simulink model "controller_sim"  (R2024a)
settings: Solver=FixedStepAuto  StartTime=0.0  StopTime=500  FixedStep=0.001  RelTol=1e-2
settings Model: Creator=filip  LastModifiedBy=raden
settings SolverCC: ZeroCrossAlgorithm=Adaptive
settings DebuggingCC: IgnoredZcDiagnostic=none

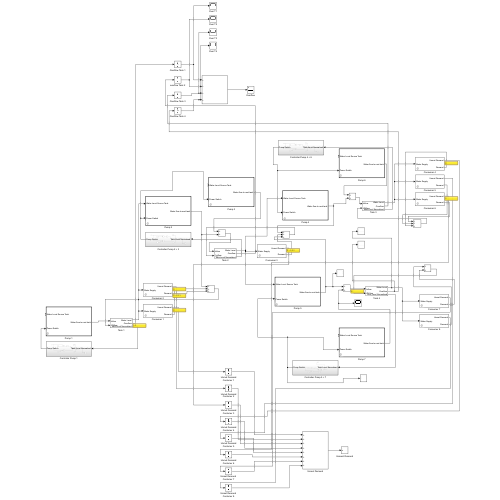
[thumbnail: Simulink's stored preview of the top-level diagram]
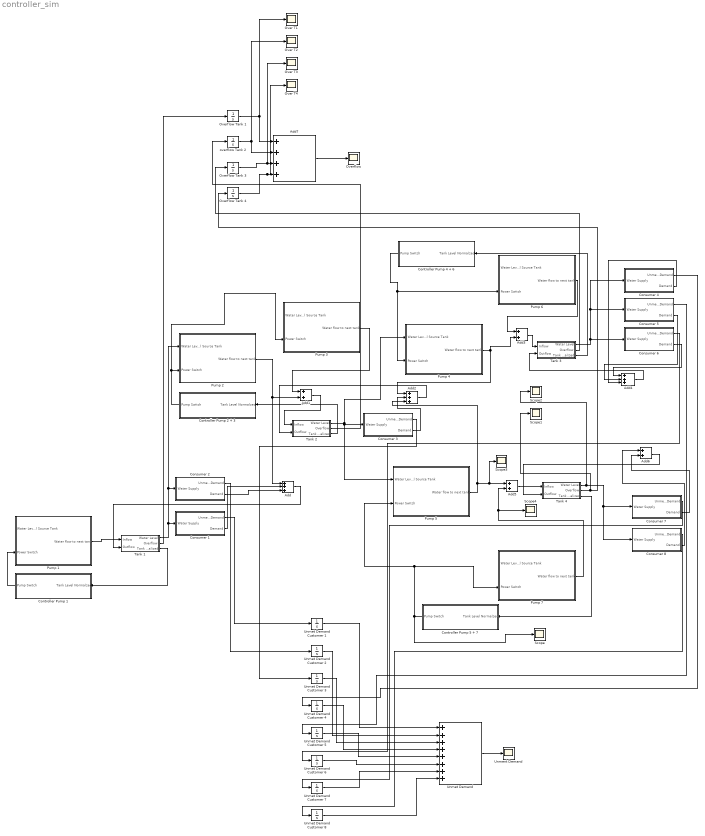
== system controller_sim ==
  Add : Sum  Inputs=+++
  Add{1,3,5..6} (4 alike) : Sum
  Add2 : Sum  Inputs=+++
  Add4 : Sum  Inputs=+++
  Add7 : Sum  Inputs=++++
  Consumer 1 : Subsystem  mask{a_i=3.0, f_i=0.4, d_i=2.0}
      mask prompts: f_i "frequenz"; d_i "delay"
  Consumer 2 : Subsystem  mask{a_i=8.0, f_i=0.6, d_i=0.5}
      mask prompts: f_i "frequenz"; d_i "delay"
  Consumer 3 : Subsystem  mask{a_i=5.0, f_i=0.2, d_i=4.0}
      mask prompts: f_i "frequenz"; d_i "delay"
  Consumer 4 : Subsystem  mask{a_i=5.0, f_i=1.0, d_i=3.0}
      mask prompts: f_i "frequenz"; d_i "delay"
  Consumer 5 : Subsystem  mask{a_i=2.0, f_i=0.4, d_i=4.0}
      mask prompts: f_i "frequenz"; d_i "delay"
  Consumer 6 : Subsystem  mask{a_i=7.0, f_i=0.1, d_i=5.0}
      mask prompts: f_i "frequenz"; d_i "delay"
  Consumer 7 : Subsystem  mask{a_i=2.0, f_i=0.9, d_i=7.0}
      mask prompts: f_i "frequenz"; d_i "delay"
  Consumer 8 : Subsystem  mask{a_i=5.0, f_i=0.6, d_i=4.0}
      mask prompts: f_i "frequenz"; d_i "delay"
  Controller Pump 1 : Subsystem
      settings: PortSchema="{\"entries\":[{\"content\":{\"sides\":[{\"content\":{\"connectorIds\":[\"Out1\"]},\"type\":\"ConnectorPlacement.EquallySpacedRectSide\",\"uuid\":\"c01aea8f-3a50-48ff-9d85-da287ef4ecfe\"},{\"content\":{\"connectorIds\":[\"In1\"],\"side\":\"RIGHT\"},\"type\":\"ConnectorPlacement.EquallySpacedRectSide\",\"uuid\":\"7272fdb4-8195-4269-b45d-955a00b5f153\"},{\"content\":{\"side\":\"TOP\"},\"type\":\"ConnectorPlacement.EquallySpacedRectSide\",\"uuid\":\"ead61a79-0064-4486-848a-5274f34ed301\"}]},\"type\":\"ConnectorPlacement.EquallySpacedConnector\",\"uuid\":\"31fbb0a2-b36d-48d4-9bb2-4bba902ab975\"}],\"packageUris\":[\"http://schema.mathworks.com/mf0/Connector/R2020b\"],\"version\":\"1.0\"}"
  Controller Pump 2 + 3 : Subsystem
      settings: PortSchema="{\"entries\":[{\"content\":{\"sides\":[{\"content\":{\"connectorIds\":[\"Out1\"]},\"type\":\"ConnectorPlacement.EquallySpacedRectSide\",\"uuid\":\"c01aea8f-3a50-48ff-9d85-da287ef4ecfe\"},{\"content\":{\"connectorIds\":[\"In1\"],\"side\":\"RIGHT\"},\"type\":\"ConnectorPlacement.EquallySpacedRectSide\",\"uuid\":\"7272fdb4-8195-4269-b45d-955a00b5f153\"},{\"content\":{\"side\":\"TOP\"},\"type\":\"ConnectorPlacement.EquallySpacedRectSide\",\"uuid\":\"ead61a79-0064-4486-848a-5274f34ed301\"}]},\"type\":\"ConnectorPlacement.EquallySpacedConnector\",\"uuid\":\"31fbb0a2-b36d-48d4-9bb2-4bba902ab975\"}],\"packageUris\":[\"http://schema.mathworks.com/mf0/Connector/R2020b\"],\"version\":\"1.0\"}"
  Controller Pump 4 + 6 : Subsystem
      settings: PortSchema="{\"entries\":[{\"content\":{\"sides\":[{\"content\":{\"connectorIds\":[\"Out1\"]},\"type\":\"ConnectorPlacement.EquallySpacedRectSide\",\"uuid\":\"c01aea8f-3a50-48ff-9d85-da287ef4ecfe\"},{\"content\":{\"connectorIds\":[\"In1\"],\"side\":\"RIGHT\"},\"type\":\"ConnectorPlacement.EquallySpacedRectSide\",\"uuid\":\"7272fdb4-8195-4269-b45d-955a00b5f153\"},{\"content\":{\"side\":\"TOP\"},\"type\":\"ConnectorPlacement.EquallySpacedRectSide\",\"uuid\":\"ead61a79-0064-4486-848a-5274f34ed301\"}]},\"type\":\"ConnectorPlacement.EquallySpacedConnector\",\"uuid\":\"31fbb0a2-b36d-48d4-9bb2-4bba902ab975\"}],\"packageUris\":[\"http://schema.mathworks.com/mf0/Connector/R2020b\"],\"version\":\"1.0\"}"
  Controller Pump 5 + 7 : Subsystem
      settings: PortSchema="{\"entries\":[{\"content\":{\"sides\":[{\"content\":{\"connectorIds\":[\"Out1\"]},\"type\":\"ConnectorPlacement.EquallySpacedRectSide\",\"uuid\":\"c01aea8f-3a50-48ff-9d85-da287ef4ecfe\"},{\"content\":{\"connectorIds\":[\"In1\"],\"side\":\"RIGHT\"},\"type\":\"ConnectorPlacement.EquallySpacedRectSide\",\"uuid\":\"7272fdb4-8195-4269-b45d-955a00b5f153\"},{\"content\":{\"side\":\"TOP\"},\"type\":\"ConnectorPlacement.EquallySpacedRectSide\",\"uuid\":\"ead61a79-0064-4486-848a-5274f34ed301\"}]},\"type\":\"ConnectorPlacement.EquallySpacedConnector\",\"uuid\":\"31fbb0a2-b36d-48d4-9bb2-4bba902ab975\"}],\"packageUris\":[\"http://schema.mathworks.com/mf0/Connector/R2020b\"],\"version\":\"1.0\"}"
  Over T{1..4} (4 alike) : Scope
  Overflow : Scope
  Overflow Tank 1 : Integrator
  Overflow Tank 3 : Integrator
  Overflow Tank 4 : Integrator
  Pump 1 : Subsystem  TreatAsAtomicUnit=on  mask{p_i=15}
      mask prompts: p_i "volume per Time (p_i)"
  Pump 2 : Subsystem  TreatAsAtomicUnit=on  mask{p_i=20}
      mask prompts: p_i "volume per Time (p_i)"
  Pump 3 : Subsystem  TreatAsAtomicUnit=on  mask{p_i=5}
      mask prompts: p_i "volume per Time (p_i)"
  Pump 4 : Subsystem  TreatAsAtomicUnit=on  mask{p_i=7}
      mask prompts: p_i "volume per Time (p_i)"
  Pump 5 : Subsystem  TreatAsAtomicUnit=on  mask{p_i=3}
      mask prompts: p_i "volume per Time (p_i)"
  Pump 6 : Subsystem  TreatAsAtomicUnit=on  mask{p_i=5}
      mask prompts: p_i "volume per Time (p_i)"
  Pump 7 : Subsystem  TreatAsAtomicUnit=on  mask{p_i=5}
      mask prompts: p_i "volume per Time (p_i)"
  Scope{,1..4} (5 alike) : Scope
  Tank 1 : Subsystem  mask{c_i=100, c_i_init=50}
      mask prompts: c_i "capacity (c_i)"; c_i_init "Init capacity (c_i_init)"
  Tank 2 : Subsystem  mask{c_i=100, c_i_init=50}
      mask prompts: c_i "capacity (c_i)"; c_i_init "Init capacity (c_i_init)"
  Tank 3 : Subsystem  mask{c_i=100, c_i_init=50}
      mask prompts: c_i "capacity (c_i)"; c_i_init "Init capacity (c_i_init)"
  Tank 4 : Subsystem  mask{c_i=100, c_i_init=0}
      mask prompts: c_i "capacity (c_i)"; c_i_init "Init capacity (c_i_init)"
  Unment Demand : Scope
  Unmet Demand : Sum  Inputs=++++++++
  Unmet Demand Customer {1..8} (8 alike) : Integrator
  overflow Tank 2 : Integrator
  wires:
  Pump 1/1(Water flow to next tank) -> Tank 1/1(Inflow)
  Add/1 -> Tank 1/2(Outflow)
  Tank 1/1(Water Level) -> Pump 2/1(Water Level Source Tank), Consumer 2/1(Water Supply), Consumer 1/1(Water Supply)
  Pump 2/1(Water flow to next tank) -> Add/1, Add1/2
  Pump 3/1(Water flow to next tank) -> Add1/1
  Add1/1 -> Tank 2/1(Inflow)
  Tank 2/1(Water Level) -> Consumer 3/1(Water Supply), Pump 5/1(Water Level Source Tank), Pump 4/1(Water Level Source Tank)
  Pump 4/1(Water flow to next tank) -> Add3/2, Add2/1
  Consumer 3/2(Demand) -> Add2/2
  Pump 5/1(Water flow to next tank) -> Add2/3, Scope3/1, Add5/1
  Add2/1 -> Tank 2/2(Outflow)
  Pump 6/1(Water flow to next tank) -> Add3/1
  Add3/1 -> Tank 3/1(Inflow)
  Tank 3/1(Water Level) -> Consumer 6/1(Water Supply), Consumer 5/1(Water Supply), Consumer 4/1(Water Supply)
  Consumer 6/2(Demand) -> Add4/1
  Consumer 5/2(Demand) -> Add4/2
  Consumer 4/2(Demand) -> Add4/3
  Add4/1 -> Tank 3/2(Outflow)
  Pump 7/1(Water flow to next tank) -> Add5/2, Scope4/1
  Add5/1 -> Tank 4/1(Inflow)
  Tank 4/1(Water Level) -> Scope2/1, Consumer 8/1(Water Supply), Consumer 7/1(Water Supply)
  Consumer 7/2(Demand) -> Add6/2
  Consumer 8/2(Demand) -> Add6/1
  Add6/1 -> Tank 4/2(Outflow)
  Consumer 2/1(Unmet Demand) -> Unmet Demand Customer 2/1
  Consumer 3/1(Unmet Demand) -> Unmet Demand Customer 3/1
  Consumer 4/1(Unmet Demand) -> Unmet Demand Customer 4/1
  Consumer 5/1(Unmet Demand) -> Unmet Demand Customer 5/1
  Consumer 6/1(Unmet Demand) -> Unmet Demand Customer 6/1
  Consumer 7/1(Unmet Demand) -> Unmet Demand Customer 7/1
  Consumer 8/1(Unmet Demand) -> Unmet Demand Customer 8/1
  Unmet Demand/1 -> Unment Demand/1
  Tank 1/2(Overflow) -> Overflow Tank 1/1
  Tank 2/2(Overflow) -> overflow Tank 2/1
  Tank 3/2(Overflow) -> Overflow Tank 3/1
  Tank 4/2(Overflow) -> Scope1/1, Overflow Tank 4/1
  Add7/1 -> Overflow/1
  Consumer 1/1(Unmet Demand) -> Unmet Demand Customer 1/1
  Consumer 1/2(Demand) -> Add/2
  Consumer 2/2(Demand) -> Add/3
  Overflow Tank 1/1 -> Over T1/1, Add7/1
  overflow Tank 2/1 -> Over T2/1, Add7/2
  Overflow Tank 3/1 -> Over T3/1, Add7/3
  Overflow Tank 4/1 -> Over T4/1, Add7/4
  Unmet Demand Customer 1/1 -> Unmet Demand/1
  Unmet Demand Customer 2/1 -> Unmet Demand/2
  Unmet Demand Customer 3/1 -> Unmet Demand/3
  Unmet Demand Customer 4/1 -> Unmet Demand/4
  Unmet Demand Customer 5/1 -> Unmet Demand/5
  Unmet Demand Customer 6/1 -> Unmet Demand/6
  Unmet Demand Customer 7/1 -> Unmet Demand/7
  Unmet Demand Customer 8/1 -> Unmet Demand/8
  Tank 1/3(Tank Level Normalized) -> Controller Pump 1/1(Tank Level Normalzed)
  Controller Pump 1/1(Pump Switch) -> Pump 1/2(Power Switch)
  Tank 2/3(Tank Level Normalized) -> Controller Pump 2 + 3/1(Tank Level Normalzed)
  Controller Pump 2 + 3/1(Pump Switch) -> Pump 2/2(Power Switch), Pump 3/2(Power Switch)
  Tank 3/3(Tank Level Normalized) -> Controller Pump 4 + 6/1(Tank Level Normalzed)
  Controller Pump 4 + 6/1(Pump Switch) -> Pump 4/2(Power Switch), Pump 6/2(Power Switch)
  Controller Pump 5 + 7/1(Pump Switch) -> Scope/1, Pump 7/2(Power Switch), Pump 5/2(Power Switch)
  Tank 4/3(Tank Level Normalized) -> Controller Pump 5 + 7/1(Tank Level Normalzed)

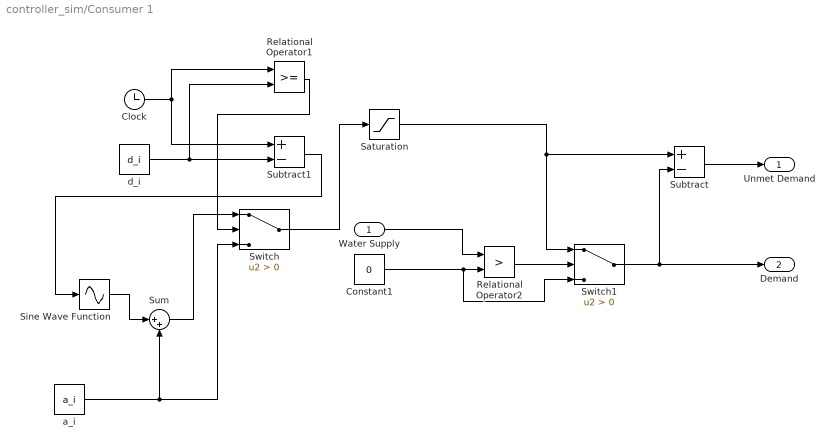
== system controller_sim/Consumer 1 ==
  Water Supply : Inport
  Clock : Clock
  Constant1 : Constant  Value=0
  Relational Operator1 : RelationalOperator  OutDataTypeStr=boolean  RndMeth=Simplest  InputSameDT=off
  Relational Operator2 : RelationalOperator  Operator=>  OutDataTypeStr=boolean  RndMeth=Simplest  InputSameDT=off
  Saturation : Saturate  UpperLimit=inf  LowerLimit=0
  Sine Wave Function : Sin  TimeSource=Use external signal  Amplitude=a_i  Frequency=f_i  SampleTime=0
  Subtract : Sum  Inputs=+-
  Subtract1 : Sum  Inputs=+-
  Sum : Sum  Inputs=|++
  Switch : Switch  Criteria=u2 > Threshold  SaturateOnIntegerOverflow=off  InputSameDT=off
  Switch1 : Switch  Criteria=u2 > Threshold  SaturateOnIntegerOverflow=off  InputSameDT=off
  a_i : Constant  Value=a_i
  d_i : Constant  Value=d_i
  Unmet Demand : Outport
  Demand : Outport  Port=2
  wires:
  a_i/1 -> Sum/2, Switch/3
  Switch/1 -> Saturation/1
  Saturation/1 -> Subtract/1, Switch1/1
  Clock/1 -> Relational Operator1/1, Subtract1/1
  d_i/1 -> Relational Operator1/2, Subtract1/2
  Subtract1/1 -> Sine Wave Function/1
  Relational Operator1/1 -> Switch/2
  Sum/1 -> Switch/1
  Sine Wave Function/1 -> Sum/1
  Water Supply/1 -> Relational Operator2/1
  Constant1/1 -> Relational Operator2/2, Switch1/3
  Relational Operator2/1 -> Switch1/2
  Switch1/1 -> Subtract/2, Demand/1
  Subtract/1 -> Unmet Demand/1

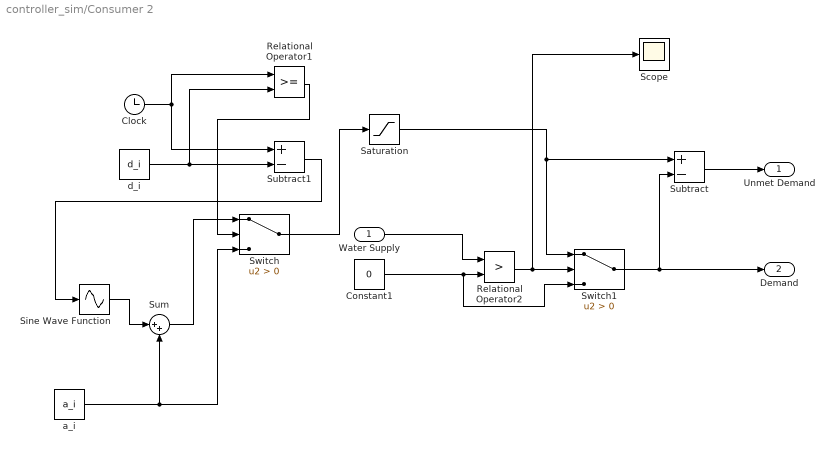
== system controller_sim/Consumer 2 ==
  Water Supply : Inport
  Clock : Clock
  Constant1 : Constant  Value=0
  Relational Operator1 : RelationalOperator  OutDataTypeStr=boolean  RndMeth=Simplest  InputSameDT=off
  Relational Operator2 : RelationalOperator  Operator=>  OutDataTypeStr=boolean  RndMeth=Simplest  InputSameDT=off
  Saturation : Saturate  UpperLimit=inf  LowerLimit=0
  Scope : Scope
  Sine Wave Function : Sin  TimeSource=Use external signal  Amplitude=a_i  Frequency=f_i  SampleTime=0
  Subtract : Sum  Inputs=+-
  Subtract1 : Sum  Inputs=+-
  Sum : Sum  Inputs=|++
  Switch : Switch  Criteria=u2 > Threshold  SaturateOnIntegerOverflow=off  InputSameDT=off
  Switch1 : Switch  Criteria=u2 > Threshold  SaturateOnIntegerOverflow=off  InputSameDT=off
  a_i : Constant  Value=a_i
  d_i : Constant  Value=d_i
  Unmet Demand : Outport
  Demand : Outport  Port=2
  wires:
  a_i/1 -> Sum/2, Switch/3
  Switch/1 -> Saturation/1
  Saturation/1 -> Subtract/1, Switch1/1
  Clock/1 -> Relational Operator1/1, Subtract1/1
  d_i/1 -> Relational Operator1/2, Subtract1/2
  Subtract1/1 -> Sine Wave Function/1
  Relational Operator1/1 -> Switch/2
  Sum/1 -> Switch/1
  Sine Wave Function/1 -> Sum/1
  Water Supply/1 -> Relational Operator2/1
  Constant1/1 -> Relational Operator2/2, Switch1/3
  Relational Operator2/1 -> Scope/1, Switch1/2
  Switch1/1 -> Subtract/2, Demand/1
  Subtract/1 -> Unmet Demand/1

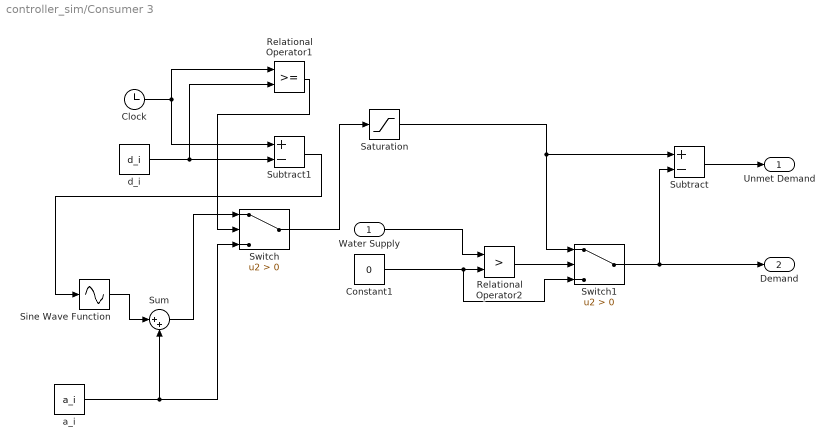
== system controller_sim/Consumer 3 ==
  Water Supply : Inport
  Clock : Clock
  Constant1 : Constant  Value=0
  Relational Operator1 : RelationalOperator  OutDataTypeStr=boolean  RndMeth=Simplest  InputSameDT=off
  Relational Operator2 : RelationalOperator  Operator=>  OutDataTypeStr=boolean  RndMeth=Simplest  InputSameDT=off
  Saturation : Saturate  UpperLimit=inf  LowerLimit=0
  Sine Wave Function : Sin  TimeSource=Use external signal  Amplitude=a_i  Frequency=f_i  SampleTime=0
  Subtract : Sum  Inputs=+-
  Subtract1 : Sum  Inputs=+-
  Sum : Sum  Inputs=|++
  Switch : Switch  Criteria=u2 > Threshold  SaturateOnIntegerOverflow=off  InputSameDT=off
  Switch1 : Switch  Criteria=u2 > Threshold  SaturateOnIntegerOverflow=off  InputSameDT=off
  a_i : Constant  Value=a_i
  d_i : Constant  Value=d_i
  Unmet Demand : Outport
  Demand : Outport  Port=2
  wires:
  a_i/1 -> Sum/2, Switch/3
  Switch/1 -> Saturation/1
  Saturation/1 -> Subtract/1, Switch1/1
  Clock/1 -> Relational Operator1/1, Subtract1/1
  d_i/1 -> Relational Operator1/2, Subtract1/2
  Subtract1/1 -> Sine Wave Function/1
  Relational Operator1/1 -> Switch/2
  Sum/1 -> Switch/1
  Sine Wave Function/1 -> Sum/1
  Water Supply/1 -> Relational Operator2/1
  Constant1/1 -> Relational Operator2/2, Switch1/3
  Relational Operator2/1 -> Switch1/2
  Switch1/1 -> Subtract/2, Demand/1
  Subtract/1 -> Unmet Demand/1

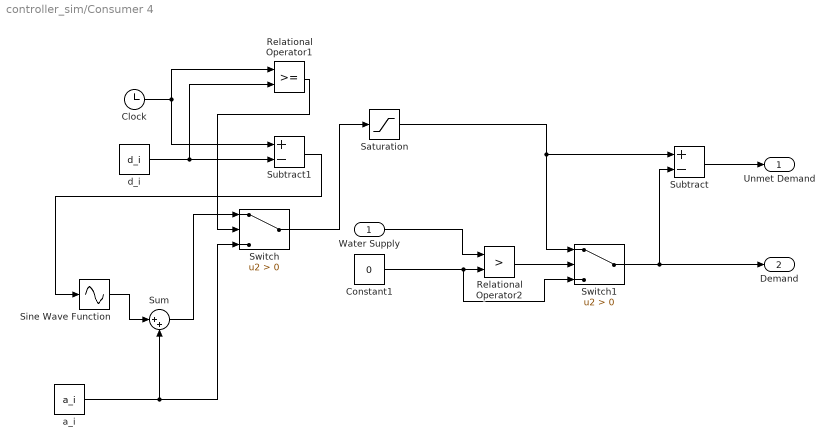
== system controller_sim/Consumer 4 ==
  Water Supply : Inport
  Clock : Clock
  Constant1 : Constant  Value=0
  Relational Operator1 : RelationalOperator  OutDataTypeStr=boolean  RndMeth=Simplest  InputSameDT=off
  Relational Operator2 : RelationalOperator  Operator=>  OutDataTypeStr=boolean  RndMeth=Simplest  InputSameDT=off
  Saturation : Saturate  UpperLimit=inf  LowerLimit=0
  Sine Wave Function : Sin  TimeSource=Use external signal  Amplitude=a_i  Frequency=f_i  SampleTime=0
  Subtract : Sum  Inputs=+-
  Subtract1 : Sum  Inputs=+-
  Sum : Sum  Inputs=|++
  Switch : Switch  Criteria=u2 > Threshold  SaturateOnIntegerOverflow=off  InputSameDT=off
  Switch1 : Switch  Criteria=u2 > Threshold  SaturateOnIntegerOverflow=off  InputSameDT=off
  a_i : Constant  Value=a_i
  d_i : Constant  Value=d_i
  Unmet Demand : Outport
  Demand : Outport  Port=2
  wires:
  a_i/1 -> Sum/2, Switch/3
  Switch/1 -> Saturation/1
  Saturation/1 -> Subtract/1, Switch1/1
  Clock/1 -> Relational Operator1/1, Subtract1/1
  d_i/1 -> Relational Operator1/2, Subtract1/2
  Subtract1/1 -> Sine Wave Function/1
  Relational Operator1/1 -> Switch/2
  Sum/1 -> Switch/1
  Sine Wave Function/1 -> Sum/1
  Water Supply/1 -> Relational Operator2/1
  Constant1/1 -> Relational Operator2/2, Switch1/3
  Relational Operator2/1 -> Switch1/2
  Switch1/1 -> Subtract/2, Demand/1
  Subtract/1 -> Unmet Demand/1

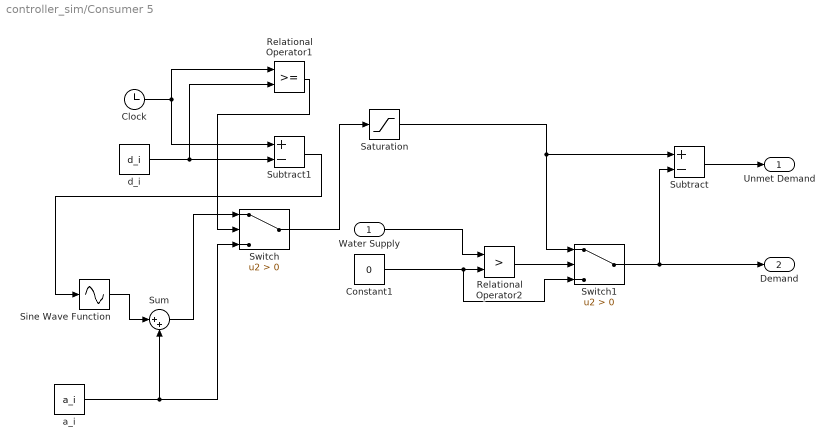
== system controller_sim/Consumer 5 ==
  Water Supply : Inport
  Clock : Clock
  Constant1 : Constant  Value=0
  Relational Operator1 : RelationalOperator  OutDataTypeStr=boolean  RndMeth=Simplest  InputSameDT=off
  Relational Operator2 : RelationalOperator  Operator=>  OutDataTypeStr=boolean  RndMeth=Simplest  InputSameDT=off
  Saturation : Saturate  UpperLimit=inf  LowerLimit=0
  Sine Wave Function : Sin  TimeSource=Use external signal  Amplitude=a_i  Frequency=f_i  SampleTime=0
  Subtract : Sum  Inputs=+-
  Subtract1 : Sum  Inputs=+-
  Sum : Sum  Inputs=|++
  Switch : Switch  Criteria=u2 > Threshold  SaturateOnIntegerOverflow=off  InputSameDT=off
  Switch1 : Switch  Criteria=u2 > Threshold  SaturateOnIntegerOverflow=off  InputSameDT=off
  a_i : Constant  Value=a_i
  d_i : Constant  Value=d_i
  Unmet Demand : Outport
  Demand : Outport  Port=2
  wires:
  a_i/1 -> Sum/2, Switch/3
  Switch/1 -> Saturation/1
  Saturation/1 -> Subtract/1, Switch1/1
  Clock/1 -> Relational Operator1/1, Subtract1/1
  d_i/1 -> Relational Operator1/2, Subtract1/2
  Subtract1/1 -> Sine Wave Function/1
  Relational Operator1/1 -> Switch/2
  Sum/1 -> Switch/1
  Sine Wave Function/1 -> Sum/1
  Water Supply/1 -> Relational Operator2/1
  Constant1/1 -> Relational Operator2/2, Switch1/3
  Relational Operator2/1 -> Switch1/2
  Switch1/1 -> Subtract/2, Demand/1
  Subtract/1 -> Unmet Demand/1

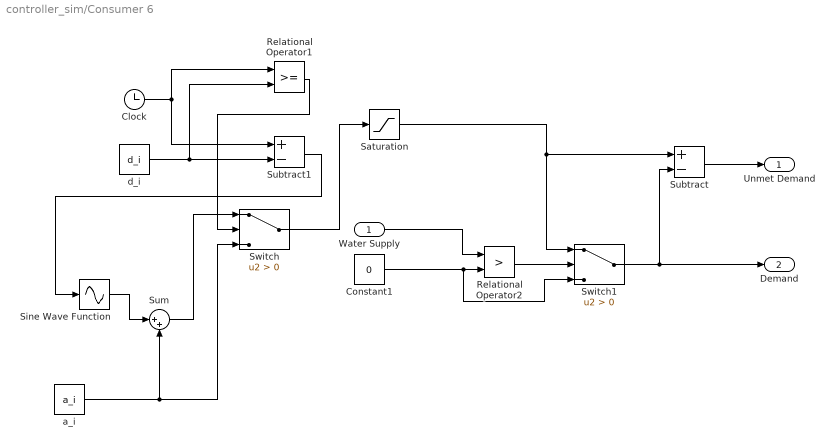
== system controller_sim/Consumer 6 ==
  Water Supply : Inport
  Clock : Clock
  Constant1 : Constant  Value=0
  Relational Operator1 : RelationalOperator  OutDataTypeStr=boolean  RndMeth=Simplest  InputSameDT=off
  Relational Operator2 : RelationalOperator  Operator=>  OutDataTypeStr=boolean  RndMeth=Simplest  InputSameDT=off
  Saturation : Saturate  UpperLimit=inf  LowerLimit=0
  Sine Wave Function : Sin  TimeSource=Use external signal  Amplitude=a_i  Frequency=f_i  SampleTime=0
  Subtract : Sum  Inputs=+-
  Subtract1 : Sum  Inputs=+-
  Sum : Sum  Inputs=|++
  Switch : Switch  Criteria=u2 > Threshold  SaturateOnIntegerOverflow=off  InputSameDT=off
  Switch1 : Switch  Criteria=u2 > Threshold  SaturateOnIntegerOverflow=off  InputSameDT=off
  a_i : Constant  Value=a_i
  d_i : Constant  Value=d_i
  Unmet Demand : Outport
  Demand : Outport  Port=2
  wires:
  a_i/1 -> Sum/2, Switch/3
  Switch/1 -> Saturation/1
  Saturation/1 -> Subtract/1, Switch1/1
  Clock/1 -> Relational Operator1/1, Subtract1/1
  d_i/1 -> Relational Operator1/2, Subtract1/2
  Subtract1/1 -> Sine Wave Function/1
  Relational Operator1/1 -> Switch/2
  Sum/1 -> Switch/1
  Sine Wave Function/1 -> Sum/1
  Water Supply/1 -> Relational Operator2/1
  Constant1/1 -> Relational Operator2/2, Switch1/3
  Relational Operator2/1 -> Switch1/2
  Switch1/1 -> Subtract/2, Demand/1
  Subtract/1 -> Unmet Demand/1

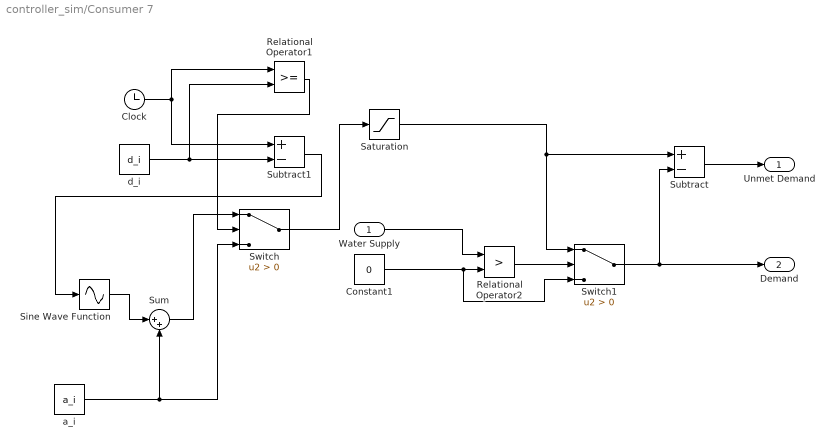
== system controller_sim/Consumer 7 ==
  Water Supply : Inport
  Clock : Clock
  Constant1 : Constant  Value=0
  Relational Operator1 : RelationalOperator  OutDataTypeStr=boolean  RndMeth=Simplest  InputSameDT=off
  Relational Operator2 : RelationalOperator  Operator=>  OutDataTypeStr=boolean  RndMeth=Simplest  InputSameDT=off
  Saturation : Saturate  UpperLimit=inf  LowerLimit=0
  Sine Wave Function : Sin  TimeSource=Use external signal  Amplitude=a_i  Frequency=f_i  SampleTime=0
  Subtract : Sum  Inputs=+-
  Subtract1 : Sum  Inputs=+-
  Sum : Sum  Inputs=|++
  Switch : Switch  Criteria=u2 > Threshold  SaturateOnIntegerOverflow=off  InputSameDT=off
  Switch1 : Switch  Criteria=u2 > Threshold  SaturateOnIntegerOverflow=off  InputSameDT=off
  a_i : Constant  Value=a_i
  d_i : Constant  Value=d_i
  Unmet Demand : Outport
  Demand : Outport  Port=2
  wires:
  a_i/1 -> Sum/2, Switch/3
  Switch/1 -> Saturation/1
  Saturation/1 -> Subtract/1, Switch1/1
  Clock/1 -> Relational Operator1/1, Subtract1/1
  d_i/1 -> Relational Operator1/2, Subtract1/2
  Subtract1/1 -> Sine Wave Function/1
  Relational Operator1/1 -> Switch/2
  Sum/1 -> Switch/1
  Sine Wave Function/1 -> Sum/1
  Water Supply/1 -> Relational Operator2/1
  Constant1/1 -> Relational Operator2/2, Switch1/3
  Relational Operator2/1 -> Switch1/2
  Switch1/1 -> Subtract/2, Demand/1
  Subtract/1 -> Unmet Demand/1

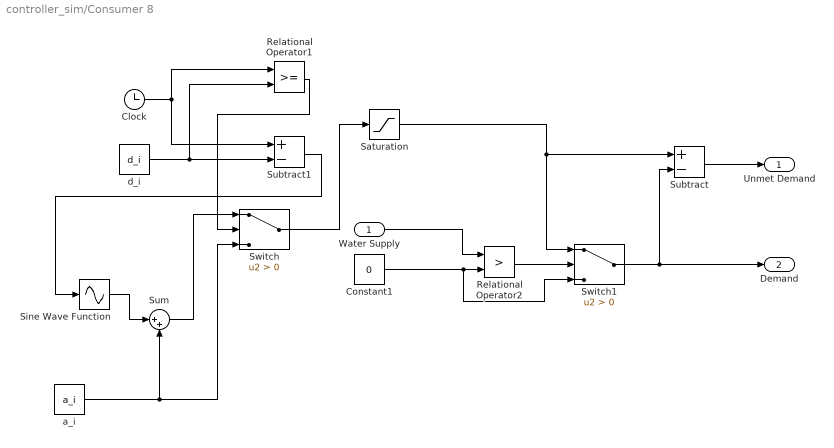
== system controller_sim/Consumer 8 ==
  Water Supply : Inport
  Clock : Clock
  Constant1 : Constant  Value=0
  Relational Operator1 : RelationalOperator  OutDataTypeStr=boolean  RndMeth=Simplest  InputSameDT=off
  Relational Operator2 : RelationalOperator  Operator=>  OutDataTypeStr=boolean  RndMeth=Simplest  InputSameDT=off
  Saturation : Saturate  UpperLimit=inf  LowerLimit=0
  Sine Wave Function : Sin  TimeSource=Use external signal  Amplitude=a_i  Frequency=f_i  SampleTime=0
  Subtract : Sum  Inputs=+-
  Subtract1 : Sum  Inputs=+-
  Sum : Sum  Inputs=|++
  Switch : Switch  Criteria=u2 > Threshold  SaturateOnIntegerOverflow=off  InputSameDT=off
  Switch1 : Switch  Criteria=u2 > Threshold  SaturateOnIntegerOverflow=off  InputSameDT=off
  a_i : Constant  Value=a_i
  d_i : Constant  Value=d_i
  Unmet Demand : Outport
  Demand : Outport  Port=2
  wires:
  a_i/1 -> Sum/2, Switch/3
  Switch/1 -> Saturation/1
  Saturation/1 -> Subtract/1, Switch1/1
  Clock/1 -> Relational Operator1/1, Subtract1/1
  d_i/1 -> Relational Operator1/2, Subtract1/2
  Subtract1/1 -> Sine Wave Function/1
  Relational Operator1/1 -> Switch/2
  Sum/1 -> Switch/1
  Sine Wave Function/1 -> Sum/1
  Water Supply/1 -> Relational Operator2/1
  Constant1/1 -> Relational Operator2/2, Switch1/3
  Relational Operator2/1 -> Switch1/2
  Switch1/1 -> Subtract/2, Demand/1
  Subtract/1 -> Unmet Demand/1

== system controller_sim/Controller Pump 1 ==
  Tank Level Normalzed : Inport
  H : RelationalOperator  Operator=>  OutDataTypeStr=boolean  RndMeth=Simplest  InputSameDT=off
  High Water Threshold : Constant  Value=0.95
  L : RelationalOperator  Operator=<  OutDataTypeStr=boolean  RndMeth=Simplest  InputSameDT=off
  Logical Operator : Logic  AllPortsSameDT=off  OutDataTypeStr=boolean
  Logical Operator1 : Logic  Operator=NOT  AllPortsSameDT=off  OutDataTypeStr=boolean
  Low Water Threshold : Constant  Value=0.5
  Pump off : Constant  Value=0
  Pump on : Constant
  Scope : Scope
  Switch : Switch  Criteria=u2 > Threshold  SaturateOnIntegerOverflow=off  InputSameDT=off
  Pump Switch : Outport
  wires:
  H/1 -> Logical Operator1/1
  Low Water Threshold/1 -> L/2
  High Water Threshold/1 -> H/2
  Tank Level Normalzed/1 -> H/1, L/1
  L/1 -> Logical Operator/2
  Logical Operator/1 -> Switch/2
  Pump off/1 -> Switch/3
  Pump on/1 -> Switch/1
  Switch/1 -> Scope/1, Pump Switch/1
  Logical Operator1/1 -> Logical Operator/1

== system controller_sim/Controller Pump 2 + 3 ==
  Tank Level Normalzed : Inport
  H : RelationalOperator  Operator=>  OutDataTypeStr=boolean  RndMeth=Simplest  InputSameDT=off
  High Water Threshold : Constant  Value=0.95
  L : RelationalOperator  Operator=<  OutDataTypeStr=boolean  RndMeth=Simplest  InputSameDT=off
  Logical Operator : Logic  AllPortsSameDT=off  OutDataTypeStr=boolean
  Logical Operator1 : Logic  Operator=NOT  AllPortsSameDT=off  OutDataTypeStr=boolean
  Low Water Threshold : Constant  Value=0.5
  Pump off : Constant  Value=0
  Pump on : Constant
  Scope : Scope
  Switch : Switch  Criteria=u2 > Threshold  SaturateOnIntegerOverflow=off  InputSameDT=off
  Pump Switch : Outport
  wires:
  H/1 -> Logical Operator1/1
  Low Water Threshold/1 -> L/2
  High Water Threshold/1 -> H/2
  Tank Level Normalzed/1 -> H/1, L/1
  L/1 -> Logical Operator/2
  Logical Operator/1 -> Switch/2
  Pump off/1 -> Switch/3
  Pump on/1 -> Switch/1
  Switch/1 -> Scope/1, Pump Switch/1
  Logical Operator1/1 -> Logical Operator/1

== system controller_sim/Controller Pump 4 + 6 ==
  Tank Level Normalzed : Inport
  H : RelationalOperator  Operator=>  OutDataTypeStr=boolean  RndMeth=Simplest  InputSameDT=off
  High Water Threshold : Constant  Value=0.95
  L : RelationalOperator  Operator=<  OutDataTypeStr=boolean  RndMeth=Simplest  InputSameDT=off
  Logical Operator : Logic  AllPortsSameDT=off  OutDataTypeStr=boolean
  Logical Operator1 : Logic  Operator=NOT  AllPortsSameDT=off  OutDataTypeStr=boolean
  Low Water Threshold : Constant  Value=0.5
  Pump off : Constant  Value=0
  Pump on : Constant
  Scope : Scope
  Switch : Switch  Criteria=u2 > Threshold  SaturateOnIntegerOverflow=off  InputSameDT=off
  Pump Switch : Outport
  wires:
  H/1 -> Logical Operator1/1
  Low Water Threshold/1 -> L/2
  High Water Threshold/1 -> H/2
  Tank Level Normalzed/1 -> H/1, L/1
  L/1 -> Logical Operator/2
  Logical Operator/1 -> Switch/2
  Pump off/1 -> Switch/3
  Pump on/1 -> Switch/1
  Switch/1 -> Scope/1, Pump Switch/1
  Logical Operator1/1 -> Logical Operator/1

== system controller_sim/Controller Pump 5 + 7 ==
  Tank Level Normalzed : Inport
  H : RelationalOperator  Operator=>  OutDataTypeStr=boolean  RndMeth=Simplest  InputSameDT=off
  High Water Threshold : Constant  Value=0.95
  L : RelationalOperator  Operator=<  OutDataTypeStr=boolean  RndMeth=Simplest  InputSameDT=off
  Logical Operator : Logic  AllPortsSameDT=off  OutDataTypeStr=boolean
  Logical Operator1 : Logic  Operator=NOT  AllPortsSameDT=off  OutDataTypeStr=boolean
  Low Water Threshold : Constant  Value=0.5
  Pump off : Constant  Value=0
  Pump on : Constant
  Scope : Scope
  Switch : Switch  Criteria=u2 > Threshold  SaturateOnIntegerOverflow=off  InputSameDT=off
  Pump Switch : Outport
  wires:
  H/1 -> Logical Operator1/1
  Low Water Threshold/1 -> L/2
  High Water Threshold/1 -> H/2
  Tank Level Normalzed/1 -> H/1, L/1
  L/1 -> Logical Operator/2
  Logical Operator/1 -> Switch/2
  Pump off/1 -> Switch/3
  Pump on/1 -> Switch/1
  Logical Operator1/1 -> Logical Operator/1
  Switch/1 -> Scope/1, Pump Switch/1

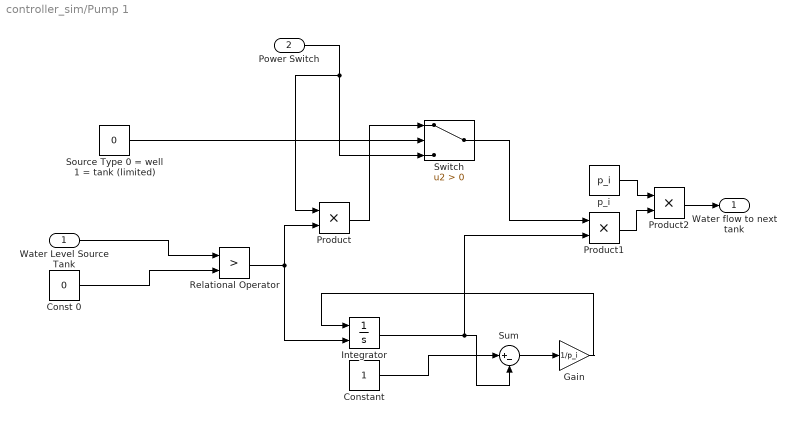
== system controller_sim/Pump 1 ==
  Water Level Source Tank : Inport
  Power Switch : Inport  Port=2
  Const 0 : Constant  Value=0
  Constant : Constant
  Gain : Gain  Gain=1/p_i
  Integrator : Integrator  ExternalReset=falling
  Product : Product
  Product1 : Product
  Product2 : Product
  Relational Operator : RelationalOperator  Operator=>  OutDataTypeStr=boolean  RndMeth=Simplest  InputSameDT=off
  Source Type 0 = well 1 = tank (limited) : Constant  Value=0
  Sum : Sum  Inputs=|+-
  Switch : Switch  Criteria=u2 > Threshold  SaturateOnIntegerOverflow=off  InputSameDT=off
  p_i : Constant  Value=p_i
  Water flow to next tank : Outport
  wires:
  Sum/1 -> Gain/1
  Integrator/1 -> Sum/2, Product1/2
  Constant/1 -> Sum/1
  Gain/1 -> Integrator/1
  Power Switch/1 -> Switch/3, Product/1
  Source Type 0 = well 1 = tank (limited)/1 -> Switch/2
  Water Level Source Tank/1 -> Relational Operator/1
  Const 0/1 -> Relational Operator/2
  Relational Operator/1 -> Integrator/2, Product/2
  Switch/1 -> Product1/1
  Product/1 -> Switch/1
  Product1/1 -> Product2/2
  p_i/1 -> Product2/1
  Product2/1 -> Water flow to next tank/1

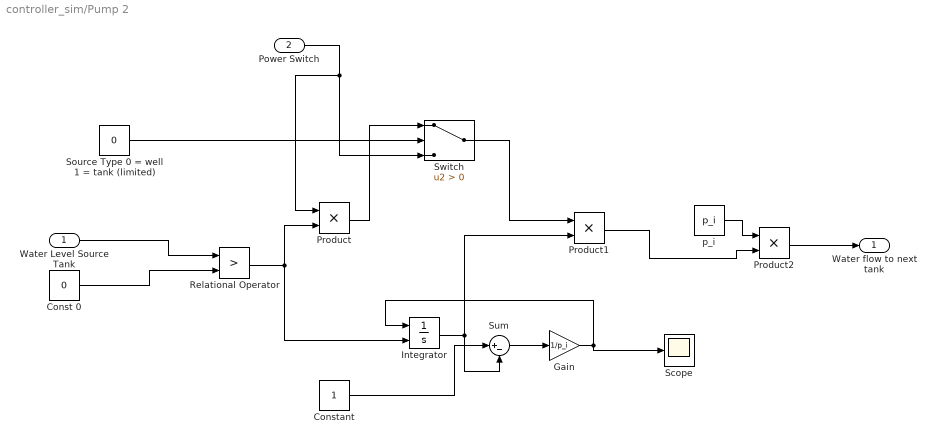
== system controller_sim/Pump 2 ==
  Water Level Source Tank : Inport
  Power Switch : Inport  Port=2
  Const 0 : Constant  Value=0
  Constant : Constant
  Gain : Gain  Gain=1/p_i
  Integrator : Integrator  ExternalReset=falling
  Product : Product
  Product1 : Product
  Product2 : Product
  Relational Operator : RelationalOperator  Operator=>  OutDataTypeStr=boolean  RndMeth=Simplest  InputSameDT=off
  Scope : Scope
  Source Type 0 = well 1 = tank (limited) : Constant  Value=0
  Sum : Sum  Inputs=|+-
  Switch : Switch  Criteria=u2 > Threshold  SaturateOnIntegerOverflow=off  InputSameDT=off
  p_i : Constant  Value=p_i
  Water flow to next tank : Outport
  wires:
  Sum/1 -> Gain/1
  Integrator/1 -> Sum/2, Product1/2
  Constant/1 -> Sum/1
  Gain/1 -> Scope/1, Integrator/1
  Power Switch/1 -> Switch/3, Product/1
  Source Type 0 = well 1 = tank (limited)/1 -> Switch/2
  Water Level Source Tank/1 -> Relational Operator/1
  Const 0/1 -> Relational Operator/2
  Relational Operator/1 -> Integrator/2, Product/2
  Switch/1 -> Product1/1
  Product/1 -> Switch/1
  p_i/1 -> Product2/1
  Product1/1 -> Product2/2
  Product2/1 -> Water flow to next tank/1

== system controller_sim/Pump 3 ==
  Water Level Source Tank : Inport
  Power Switch : Inport  Port=2
  Const 0 : Constant  Value=0
  Constant : Constant
  Gain : Gain  Gain=1/p_i
  Integrator : Integrator  ExternalReset=falling
  Product : Product
  Product1 : Product
  Product2 : Product
  Relational Operator : RelationalOperator  Operator=>  OutDataTypeStr=boolean  RndMeth=Simplest  InputSameDT=off
  Source Type 0 = well 1 = tank (limited) : Constant
  Sum : Sum  Inputs=|+-
  Switch : Switch  Criteria=u2 > Threshold  SaturateOnIntegerOverflow=off  InputSameDT=off
  p_i : Constant  Value=p_i
  Water flow to next tank : Outport
  wires:
  Sum/1 -> Gain/1
  Integrator/1 -> Sum/2, Product1/2
  Constant/1 -> Sum/1
  Gain/1 -> Integrator/1
  Power Switch/1 -> Switch/3, Product/1
  Source Type 0 = well 1 = tank (limited)/1 -> Switch/2
  Water Level Source Tank/1 -> Relational Operator/1
  Const 0/1 -> Relational Operator/2
  Relational Operator/1 -> Integrator/2, Product/2
  Switch/1 -> Product1/1
  Product/1 -> Switch/1
  p_i/1 -> Product2/1
  Product1/1 -> Product2/2
  Product2/1 -> Water flow to next tank/1

== system controller_sim/Pump 4 ==
  Water Level Source Tank : Inport
  Power Switch : Inport  Port=2
  Const 0 : Constant  Value=0
  Constant : Constant
  Gain : Gain  Gain=1/p_i
  Integrator : Integrator  ExternalReset=falling
  Product : Product
  Product1 : Product
  Product2 : Product
  Relational Operator : RelationalOperator  Operator=>  OutDataTypeStr=boolean  RndMeth=Simplest  InputSameDT=off
  Source Type 0 = well 1 = tank (limited) : Constant  Value=0
  Sum : Sum  Inputs=|+-
  Switch : Switch  Criteria=u2 > Threshold  SaturateOnIntegerOverflow=off  InputSameDT=off
  p_i : Constant  Value=p_i
  Water flow to next tank : Outport
  wires:
  Sum/1 -> Gain/1
  Integrator/1 -> Sum/2, Product1/2
  Constant/1 -> Sum/1
  Gain/1 -> Integrator/1
  Power Switch/1 -> Switch/3, Product/1
  Source Type 0 = well 1 = tank (limited)/1 -> Switch/2
  Water Level Source Tank/1 -> Relational Operator/1
  Const 0/1 -> Relational Operator/2
  Relational Operator/1 -> Integrator/2, Product/2
  Switch/1 -> Product1/1
  Product/1 -> Switch/1
  p_i/1 -> Product2/1
  Product1/1 -> Product2/2
  Product2/1 -> Water flow to next tank/1

== system controller_sim/Pump 5 ==
  Water Level Source Tank : Inport
  Power Switch : Inport  Port=2
  Const 0 : Constant  Value=0
  Constant : Constant
  Gain : Gain  Gain=1/p_i
  Integrator : Integrator  ExternalReset=falling
  Product : Product
  Product1 : Product
  Product2 : Product
  Relational Operator : RelationalOperator  Operator=>  OutDataTypeStr=boolean  RndMeth=Simplest  InputSameDT=off
  Source Type 0 = well 1 = tank (limited) : Constant  Value=0
  Sum : Sum  Inputs=|+-
  Switch : Switch  Criteria=u2 > Threshold  SaturateOnIntegerOverflow=off  InputSameDT=off
  p_i : Constant  Value=p_i
  Water flow to next tank : Outport
  wires:
  Sum/1 -> Gain/1
  Integrator/1 -> Sum/2, Product1/2
  Constant/1 -> Sum/1
  Gain/1 -> Integrator/1
  Power Switch/1 -> Switch/3, Product/1
  Source Type 0 = well 1 = tank (limited)/1 -> Switch/2
  Water Level Source Tank/1 -> Relational Operator/1
  Const 0/1 -> Relational Operator/2
  Relational Operator/1 -> Integrator/2, Product/2
  Switch/1 -> Product1/1
  Product/1 -> Switch/1
  p_i/1 -> Product2/1
  Product2/1 -> Water flow to next tank/1
  Product1/1 -> Product2/2

== system controller_sim/Pump 6 ==
  Water Level Source Tank : Inport
  Power Switch : Inport  Port=2
  Const 0 : Constant  Value=0
  Constant : Constant
  Gain : Gain  Gain=1/p_i
  Integrator : Integrator  ExternalReset=falling
  Product : Product
  Product1 : Product
  Product2 : Product
  Relational Operator : RelationalOperator  Operator=>  OutDataTypeStr=boolean  RndMeth=Simplest  InputSameDT=off
  Source Type 0 = well 1 = tank (limited) : Constant  Value=0
  Sum : Sum  Inputs=|+-
  Switch : Switch  Criteria=u2 > Threshold  SaturateOnIntegerOverflow=off  InputSameDT=off
  p_i : Constant  Value=p_i
  Water flow to next tank : Outport
  wires:
  Sum/1 -> Gain/1
  Integrator/1 -> Sum/2, Product1/2
  Constant/1 -> Sum/1
  Gain/1 -> Integrator/1
  Power Switch/1 -> Switch/3, Product/1
  Source Type 0 = well 1 = tank (limited)/1 -> Switch/2
  Water Level Source Tank/1 -> Relational Operator/1
  Const 0/1 -> Relational Operator/2
  Relational Operator/1 -> Integrator/2, Product/2
  Switch/1 -> Product1/1
  Product/1 -> Switch/1
  p_i/1 -> Product2/1
  Product1/1 -> Product2/2
  Product2/1 -> Water flow to next tank/1

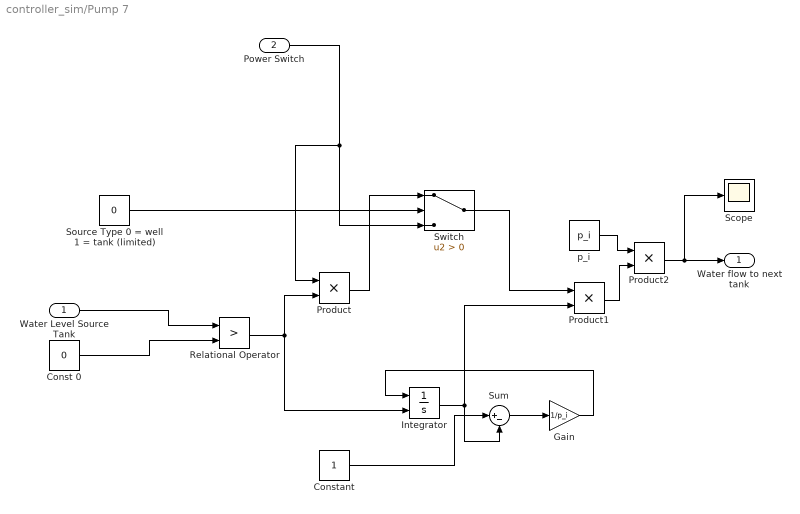
== system controller_sim/Pump 7 ==
  Water Level Source Tank : Inport
  Power Switch : Inport  Port=2
  Const 0 : Constant  Value=0
  Constant : Constant
  Gain : Gain  Gain=1/p_i
  Integrator : Integrator  ExternalReset=falling
  Product : Product
  Product1 : Product
  Product2 : Product
  Relational Operator : RelationalOperator  Operator=>  OutDataTypeStr=boolean  RndMeth=Simplest  InputSameDT=off
  Scope : Scope
  Source Type 0 = well 1 = tank (limited) : Constant  Value=0
  Sum : Sum  Inputs=|+-
  Switch : Switch  Criteria=u2 > Threshold  SaturateOnIntegerOverflow=off  InputSameDT=off
  p_i : Constant  Value=p_i
  Water flow to next tank : Outport
  wires:
  Sum/1 -> Gain/1
  Integrator/1 -> Sum/2, Product1/2
  Constant/1 -> Sum/1
  Gain/1 -> Integrator/1
  Power Switch/1 -> Switch/3, Product/1
  Source Type 0 = well 1 = tank (limited)/1 -> Switch/2
  Water Level Source Tank/1 -> Relational Operator/1
  Const 0/1 -> Relational Operator/2
  Relational Operator/1 -> Integrator/2, Product/2
  Switch/1 -> Product1/1
  Product/1 -> Switch/1
  p_i/1 -> Product2/1
  Product1/1 -> Product2/2
  Product2/1 -> Scope/1, Water flow to next tank/1

== system controller_sim/Tank 1 ==
  Inflow : Inport
  Outflow : Inport  Port=2
  Capacity c_i : Constant  Value=c_i
  Divide : Product  Inputs=*/
  Gain : Gain
  "Initial Waterlevel c_i, init" : Constant  Value=c_i_init
  Integrator : Integrator  InitialConditionSource=external
  Product : Product
  Relational Operator : RelationalOperator  Operator=>  OutDataTypeStr=boolean  RndMeth=Simplest  InputSameDT=off
  Saturation : Saturate  UpperLimit=100  LowerLimit=0
  Subtract : Sum  Inputs=+-
  Sum : Sum  Inputs=|+-
  Water Level : Outport
  Overflow : Outport  Port=2
  Tank Level Normalized : Outport  Port=3
  wires:
  Inflow/1 -> Sum/1
  Outflow/1 -> Sum/2
  Sum/1 -> Integrator/1
  Integrator/1 -> Gain/1
  Gain/1 -> Relational Operator/1, Subtract/1, Saturation/1
  Capacity c_i/1 -> Relational Operator/2, Subtract/2, Divide/2
  Saturation/1 -> Divide/1, Water Level/1
  Product/1 -> Overflow/1
  Subtract/1 -> Product/1
  Relational Operator/1 -> Product/2
  "Initial Waterlevel c_i, init"/1 -> Integrator/2
  Divide/1 -> Tank Level Normalized/1

== system controller_sim/Tank 2 ==
  Inflow : Inport
  Outflow : Inport  Port=2
  Capacity c_i : Constant  Value=c_i
  Divide : Product  Inputs=*/
  Gain : Gain
  "Initial Waterlevel c_i, init" : Constant  Value=c_i_init
  Integrator : Integrator  InitialConditionSource=external
  Product : Product
  Relational Operator : RelationalOperator  Operator=>  OutDataTypeStr=boolean  RndMeth=Simplest  InputSameDT=off
  Saturation : Saturate  UpperLimit=100  LowerLimit=0
  Subtract : Sum  Inputs=+-
  Sum : Sum  Inputs=|+-
  Water Level : Outport
  Overflow : Outport  Port=2
  Tank Level Normalized : Outport  Port=3
  wires:
  Inflow/1 -> Sum/1
  Outflow/1 -> Sum/2
  Sum/1 -> Integrator/1
  Integrator/1 -> Gain/1
  Gain/1 -> Relational Operator/1, Subtract/1, Saturation/1
  Capacity c_i/1 -> Relational Operator/2, Subtract/2, Divide/2
  Saturation/1 -> Divide/1, Water Level/1
  Product/1 -> Overflow/1
  Subtract/1 -> Product/1
  Relational Operator/1 -> Product/2
  "Initial Waterlevel c_i, init"/1 -> Integrator/2
  Divide/1 -> Tank Level Normalized/1

== system controller_sim/Tank 3 ==
  Inflow : Inport
  Outflow : Inport  Port=2
  Capacity c_i : Constant  Value=c_i
  Divide : Product  Inputs=*/
  Gain : Gain
  "Initial Waterlevel c_i, init" : Constant  Value=c_i_init
  Integrator : Integrator  InitialConditionSource=external
  Product : Product
  Relational Operator : RelationalOperator  Operator=>  OutDataTypeStr=boolean  RndMeth=Simplest  InputSameDT=off
  Saturation : Saturate  UpperLimit=100  LowerLimit=0
  Subtract : Sum  Inputs=+-
  Sum : Sum  Inputs=|+-
  Water Level : Outport
  Overflow : Outport  Port=2
  Tank Level Normalized : Outport  Port=3
  wires:
  Inflow/1 -> Sum/1
  Outflow/1 -> Sum/2
  Sum/1 -> Integrator/1
  Integrator/1 -> Gain/1
  Gain/1 -> Relational Operator/1, Subtract/1, Saturation/1
  Capacity c_i/1 -> Relational Operator/2, Subtract/2, Divide/2
  Saturation/1 -> Divide/1, Water Level/1
  Product/1 -> Overflow/1
  Subtract/1 -> Product/1
  Relational Operator/1 -> Product/2
  "Initial Waterlevel c_i, init"/1 -> Integrator/2
  Divide/1 -> Tank Level Normalized/1

== system controller_sim/Tank 4 ==
  Inflow : Inport
  Outflow : Inport  Port=2
  Capacity c_i : Constant  Value=c_i
  Divide : Product  Inputs=*/
  Gain : Gain
  "Initial Waterlevel c_i, init" : Constant  Value=c_i_init
  Integrator : Integrator  InitialConditionSource=external
  Product : Product
  Relational Operator : RelationalOperator  Operator=>  OutDataTypeStr=boolean  RndMeth=Simplest  InputSameDT=off
  Saturation : Saturate  UpperLimit=100  LowerLimit=0
  Subtract : Sum  Inputs=+-
  Sum : Sum  Inputs=|+-
  Water Level : Outport
  Overflow : Outport  Port=2
  Tank Level Normalized : Outport  Port=3
  wires:
  Inflow/1 -> Sum/1
  Outflow/1 -> Sum/2
  Sum/1 -> Integrator/1
  Integrator/1 -> Gain/1
  Gain/1 -> Relational Operator/1, Subtract/1, Saturation/1
  Capacity c_i/1 -> Relational Operator/2, Divide/2, Subtract/2
  Saturation/1 -> Divide/1, Water Level/1
  Subtract/1 -> Product/1
  Relational Operator/1 -> Product/2
  "Initial Waterlevel c_i, init"/1 -> Integrator/2
  Product/1 -> Overflow/1
  Divide/1 -> Tank Level Normalized/1
